simulink model "Lab1B_Task2"  (R2019b)
settings: Solver=FixedStepAuto  StartTime=0.0  StopTime=50.0  FixedStep=1e-1  RelTol=1e-3
settings Model: Creator=sinow  LastModifiedBy=sinow

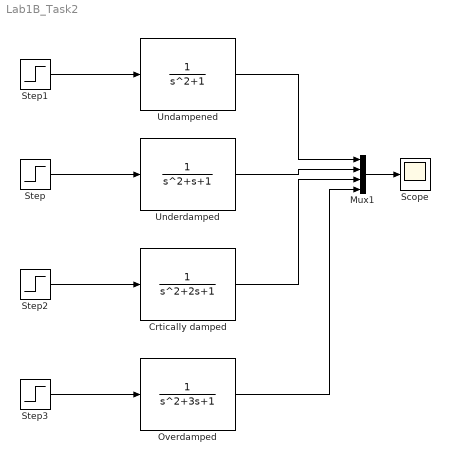
== system Lab1B_Task2 ==
  Crtically damped : TransferFcn
  Mux1 : Mux
  Overdamped : TransferFcn  Denominator=[1 3 1]
  Scope : Scope
  Step{,1..3} (4 alike) : Step  Time=0  SampleTime=0
  Undampened : TransferFcn  Denominator=[1 0 1]
  Underdamped : TransferFcn  Denominator=[1 1 1]
  wires:
  Step/1 -> Underdamped/1
  Underdamped/1 -> Mux1/2
  Undampened/1 -> Mux1/1
  Step1/1 -> Undampened/1
  Crtically damped/1 -> Mux1/3
  Step2/1 -> Crtically damped/1
  Overdamped/1 -> Mux1/4
  Step3/1 -> Overdamped/1
  Mux1/1 -> Scope/1
